simulink subsystem "Vehicle_Model"  (R2022b)
settings: Solver=VariableStepAuto  StartTime=0.0  StopTime=10.0  RelTol=1e-3
undefined symbols (not defined in the file): chassis, dZ, F0z, IMU_accel, IMU_gyro, IMU_mag, phi, powertrain, psi, sim, sus, suspension, theta, trn, veh, VEH, whl, X, Xdot, Y, Ydot, Z, Zdot
libraries: fl_lib x53, nesl_utility x15, vehdynlibtire x10, vehdynlibsuspension x8, EngineCoolingComponents_lib x5, autolibutils x5, sharedtransform x5, shared6dof x2, sensorgpslib x1, mspsensorlib x1, dspstat3 x1, SimscapeFluids_lib x1
(part 1 of 8)
settings Model: Creator=Inver  LastModifiedBy=Inver

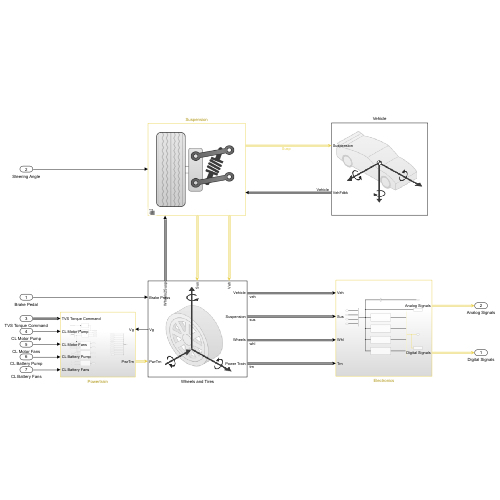
[thumbnail: Simulink's stored preview of the top-level diagram]
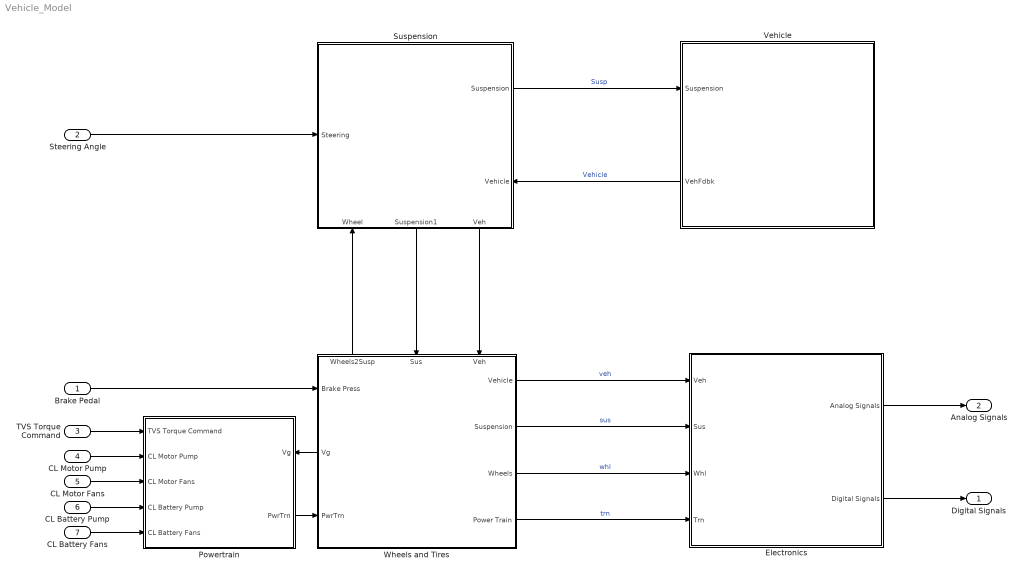
== system Vehicle_Model ==
  Brake Pedal : Inport
  Steering Angle : Inport  Port=2
  TVS Torque Command : Inport  Port=3
  CL Motor Pump : Inport  Port=4
  CL Motor Fans : Inport  Port=5
  CL Battery Pump : Inport  Port=6
  CL Battery Fans : Inport  Port=7
  Electronics : Subsystem
  Powertrain : Subsystem
      settings: PortSchema="{\"entries\":[{\"content\":{\"sides\":[{\"content\":{\"connectorIds\":[\"In1\",\"In2\",\"In3\",\"In4\",\"In5\"]},\"type\":\"ConnectorPlacement.EquallySpacedRectSide\",\"uuid\":\"895a90fc-946f-4344-af69-c005acf2f614\"},{\"content\":{\"connectorIds\":[\"In6\",\"Out1\"],\"side\":\"RIGHT\"},\"type\":\"ConnectorPlacement.EquallySpacedRectSide\",\"uuid\":\"931fcb49-b75e-480c-a4d6-2f82b080d057\"},{\"content\":{\"connectorIds\":[],\"side\":\"TOP\"},\"type\":\"ConnectorPlacement.EquallySpacedRectSide\",\"uuid\":\"d1b12b51-387e-4553-b5da-149d57232505\"}]},\"type\":\"ConnectorPlacement.EquallySpacedConnector\",\"uuid\":\"0cb2c3dd-4627-421c-9ed4-7e8c572a9937\"}],\"packageUris\":[\"http://schema.mathworks.com/mf0/Connector/R2020b\"],\"version\":\"1.0\"}"
  Suspension : Subsystem  Variant=on  VariantControlMode=label  LabelModeActiveChoice=1
      settings: PortSchema="{\"entries\":[{\"content\":{\"sides\":[{\"content\":{\"connectorIds\":[\"In1\"]},\"type\":\"ConnectorPlacement.EquallySpacedRectSide\",\"uuid\":\"d90bf910-501d-4dd1-a367-d76bd42ab174\"},{\"content\":{\"connectorIds\":[\"Out1\",\"In3\"],\"side\":\"RIGHT\"},\"type\":\"ConnectorPlacement.EquallySpacedRectSide\",\"uuid\":\"1fe7da07-1086-4d5e-8baf-d5d069455d6e\"},{\"content\":{\"connectorIds\":[],\"side\":\"TOP\"},\"type\":\"ConnectorPlacement.EquallySpacedRectSide\",\"uuid\":\"6ff63b9e-45bb-47e9-90cd-47f8e0815e57\"},{\"content\":{\"connectorIds\":[\"In2\",\"Out2\",\"Out3\"],\"side\":\"BOTTOM\"},\"type\":\"ConnectorPlacement.EquallySpacedRectSide\",\"uuid\":\"116c6de0-7bfa-4dc1-bfd0-57a2fffb3aa0\"}]},\"type\":\"ConnectorPlacement.EquallySpacedConnector\",\"uuid\":\"6475b998-12b0-4b0e-8a20-c379b8e08c7c\"}],\"packageUris\":[\"http://schema.mathworks.com/mf0/Connector/R2020b\"],\"version\":\"1.0\"}"
      mask Display:
      | switch str2num(get_param(gcb,'ActiveVariant'))
      |     case 1
      |         image('suspdw.png');
      |     case 2
      |         image([imread('suspindmap.png');imread('suspsamap.png')]);
      |     case 3
      |          image([imread('suspmacp.png');imread('suspsacoil.png')]);
      |     case 4
      |          image('suspmacp.png');
      |     case 5
      |          image('suspindmap.png');
      |     case 6
      |          image('suspkandc.png');
      | end
  Vehicle : Subsystem
      settings: PortSchema="{\"entries\":[{\"content\":{\"sides\":[{\"content\":{\"connectorIds\":[\"In1\",\"Out1\"]},\"type\":\"ConnectorPlacement.EquallySpacedRectSide\",\"uuid\":\"63fa377f-0583-4c60-bac7-9bd73dadd9a1\"},{\"content\":{\"connectorIds\":[],\"side\":\"RIGHT\"},\"type\":\"ConnectorPlacement.EquallySpacedRectSide\",\"uuid\":\"7f668e34-aa5e-4f2f-9be8-80fbb83ff2c8\"},{\"content\":{\"connectorIds\":[],\"side\":\"TOP\"},\"type\":\"ConnectorPlacement.EquallySpacedRectSide\",\"uuid\":\"511f439c-568f-45f1-9ff4-54e644eb8180\"}]},\"type\":\"ConnectorPlacement.EquallySpacedConnector\",\"uuid\":\"b54bf87e-fa06-468b-8fa9-38148d60ed3d\"}],\"packageUris\":[\"http://schema.mathworks.com/mf0/Connector/R2020b\"],\"version\":\"1.0\"}"
      mask Display: image('6dofcar.png');
  Wheels and Tires : Subsystem
      settings: PortSchema="{\"entries\":[{\"content\":{\"sides\":[{\"content\":{\"connectorIds\":[\"In1\",\"Out6\",\"In2\"]},\"type\":\"ConnectorPlacement.EquallySpacedRectSide\",\"uuid\":\"77263124-783e-4307-b979-a6212540af24\"},{\"content\":{\"connectorIds\":[\"Out1\",\"Out2\",\"Out3\",\"Out4\"],\"side\":\"RIGHT\"},\"type\":\"ConnectorPlacement.EquallySpacedRectSide\",\"uuid\":\"cb03b446-69c2-4dbf-929b-d33818acfe8b\"},{\"content\":{\"connectorIds\":[\"Out5\",\"In3\",\"In4\"],\"side\":\"TOP\"},\"type\":\"ConnectorPlacement.EquallySpacedRectSide\",\"uuid\":\"8e7e4023-62e5-48a8-8666-b4c8bb14cd01\"}]},\"type\":\"ConnectorPlacement.EquallySpacedConnector\",\"uuid\":\"1061f0db-ec8e-49bd-8d66-b4a53eaeacfa\"}],\"packageUris\":[\"http://schema.mathworks.com/mf0/Connector/R2020b\"],\"version\":\"1.0\"}"
      mask Display: image('wheel3dof.png')
  Digital Signals : Outport  PortDimensions={292}
  Analog Signals : Outport  Port=2  PortDimensions={292}
  wires:
  CL Motor Pump/1 -> Powertrain/2(CL Motor Pump)
  CL Motor Fans/1 -> Powertrain/3(CL Motor Fans)
  Wheels and Tires/1(Vehicle) -> Electronics/1(Veh)  "veh"
  Wheels and Tires/6(Vg) -> Powertrain/6(Vg)
  CL Battery Pump/1 -> Powertrain/4(CL Battery Pump)
  Electronics/2(Digital Signals) -> Digital Signals/1
  CL Battery Fans/1 -> Powertrain/5(CL Battery Fans)
  Vehicle/1(VehFdbk) -> Suspension/3(Vehicle)  "Vehicle"
  Suspension/2(Suspension1) -> Wheels and Tires/3(Sus)
  TVS Torque Command/1 -> Powertrain/1(TVS Torque Command)
  Steering Angle/1 -> Suspension/1(Steering)
  Electronics/1(Analog Signals) -> Analog Signals/1
  Wheels and Tires/5(Wheels2Susp) -> Suspension/2(Wheel)
  Brake Pedal/1 -> Wheels and Tires/1(Brake Press)
  Wheels and Tires/2(Suspension) -> Electronics/2(Sus)  "sus"
  Suspension/1(Suspension) -> Vehicle/1(Suspension)  "Susp"
  Suspension/3(Veh) -> Wheels and Tires/4(Veh)
  Powertrain/1(PwrTrn) -> Wheels and Tires/2(PwrTrn)
  Wheels and Tires/3(Wheels) -> Electronics/3(Whl)  "whl"
  Wheels and Tires/4(Power Train) -> Electronics/4(Trn)  "trn"

== system Vehicle_Model/Electronics ==
  Veh : Inport
  Sus : Inport  Port=2
  Whl : Inport  Port=3
  Trn : Inport  Port=4
  All Veh Info : BusCreator  Inputs=veh,sus,whl,trn
  Bus Selector2 : BusSelector  OutputSignals=veh.InertFrm.Cg.Disp,veh.InertFrm.Cg.Ang.psi,veh.BdyFrm.Cg.Vel,veh.BdyFrm.Cg.AngVel.r,sus.Sus.steering_angle,whl.TireFrame.Omega,whl.TireFrame.GndFz  OutputAsBus=on
  Cooling Sensors : Subsystem
  Corner Dynamics Sensors : Subsystem
  Digital SIgnals : BusCreator  Inputs=4
  Navigation Sensors : Subsystem
  Power Sensors : Subsystem
  To Workspace : ToWorkspace  VariableName=Digital_Signals  SaveFormat=Timeseries  SampleTime=-1
  To Workspace1 : ToWorkspace  VariableName=Vehicle_Signals  SaveFormat=Timeseries  SampleTime=-1
  Analog Signals : Outport
  Digital Signals : Outport  Port=2
  wires:
  Sus/1 -> All Veh Info/2
  Whl/1 -> All Veh Info/3
  Trn/1 -> All Veh Info/4
  Bus Selector2/1 -> Analog Signals/1
  Navigation Sensors/1(Navigation Sensors) -> Digital SIgnals/1  "Navigation Sensors"
  Power Sensors/1(Power Sensors) -> Digital SIgnals/2  "Power Sensors"
  Corner Dynamics Sensors/1(Corner Dynamics Sensors) -> Digital SIgnals/4  "Corner Dynamics Sensors"
  Digital SIgnals/1 -> Digital Signals/1, To Workspace/1  "Digital Signls"
  Cooling Sensors/1(Cooling Sensors) -> Digital SIgnals/3  "Cooling Sensors"
  All Veh Info/1 -> Bus Selector2/1, To Workspace1/1, Navigation Sensors/1(Analog Signals), Corner Dynamics Sensors/1(Analog Signals), Cooling Sensors/1(Analog Signals), Power Sensors/1(Analog Signals)
  Veh/1 -> All Veh Info/1  "veh"

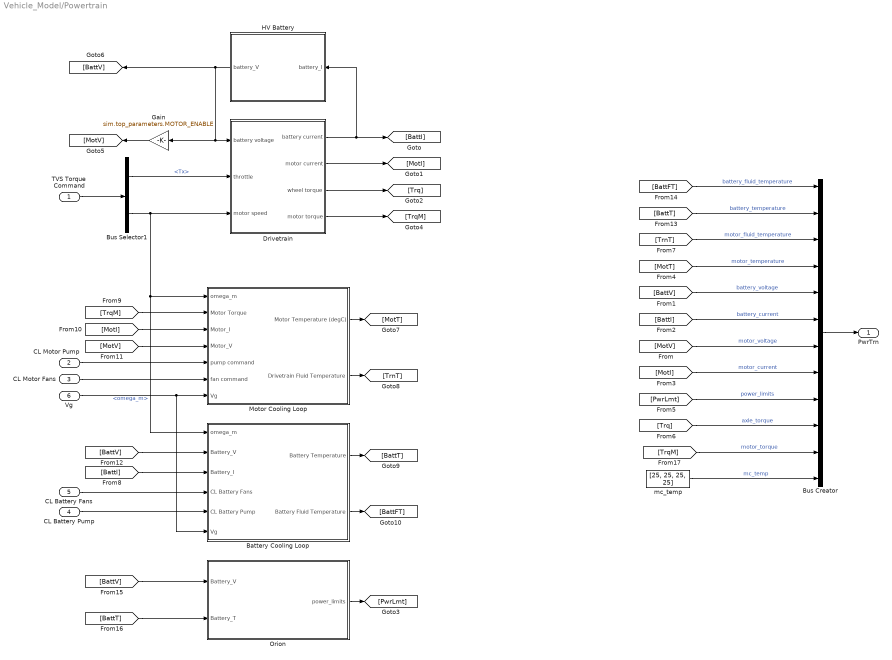
== system Vehicle_Model/Powertrain ==
  TVS Torque Command : Inport
  CL Motor Pump : Inport  Port=2
  CL Motor Fans : Inport  Port=3
  CL Battery Pump : Inport  Port=4
  CL Battery Fans : Inport  Port=5
  Vg : Inport  Port=6
  Battery Cooling Loop : Subsystem
  Bus Creator : BusCreator  Inputs=12
  Bus Selector1 : BusSelector  OutputSignals=Tx,omega_m
  Drivetrain : Subsystem
  Gain : Gain  Gain=sim.top_parameters.MOTOR_ENABLE
  HV Battery : Subsystem
  Motor Cooling Loop : Subsystem
  Orion : Subsystem
  mc_temp : Constant  Value=[25, 25, 25, 25]
  PwrTrn : Outport
  wires:
  Drivetrain/3(wheel torque) -> [Trq]
  [BattT] -> Orion/2(Battery_T)
  [Trq] -> Bus Creator/10  "axle_torque"
  [TrnT] -> Bus Creator/3  "motor_fluid_temperature"
  Vg/1 -> Motor Cooling Loop/7(Vg), Battery Cooling Loop/6(Vg)
  CL Battery Fans/1 -> Battery Cooling Loop/4(CL Battery Fans)
  [MotT] -> Bus Creator/4  "motor_temperature"
  Battery Cooling Loop/2(Battery Fluid Temperature) -> [BattFT]
  [BattI] -> Bus Creator/6  "battery_current"
  [MotI] -> Bus Creator/8  "motor_current"
  [MotV] -> Motor Cooling Loop/4(Motor_V)
  Motor Cooling Loop/2(Drivetrain Fluid Temperature) -> [TrnT]
  CL Battery Pump/1 -> Battery Cooling Loop/5(CL Battery Pump)
  Bus Selector1/2 -> Drivetrain/3(motor speed), Motor Cooling Loop/1(omega_m), Battery Cooling Loop/1(omega_m)  "<omega_m>"
  Bus Selector1/1 -> Drivetrain/2(throttle)  "<Tx>"
  CL Motor Pump/1 -> Motor Cooling Loop/5(pump command)
  Battery Cooling Loop/1(Battery Temperature) -> [BattT]
  [BattI] -> Battery Cooling Loop/3(Battery_I)
  [BattV] -> Orion/1(Battery_V)
  Motor Cooling Loop/1(Motor Temperature (degC)) -> [MotT]
  HV Battery/1(battery_V) -> [BattV], Gain/1, Drivetrain/1(battery voltage)
  [MotV] -> Bus Creator/7  "motor_voltage"
  [BattV] -> Bus Creator/5  "battery_voltage"
  [MotI] -> Motor Cooling Loop/3(Motor_I)
  [BattV] -> Battery Cooling Loop/2(Battery_V)
  [BattFT] -> Bus Creator/1  "battery_fluid_temperature"
  Drivetrain/1(battery current) -> HV Battery/1(battery_I), [BattI]
  Bus Creator/1 -> PwrTrn/1
  CL Motor Fans/1 -> Motor Cooling Loop/6(fan command)
  [PwrLmt] -> Bus Creator/9  "power_limits"
  [BattT] -> Bus Creator/2  "battery_temperature"
  Orion/1(power_limits) -> [PwrLmt]
  [TrqM] -> Motor Cooling Loop/2(Motor Torque)
  mc_temp/1 -> Bus Creator/12  "mc_temp"
  TVS Torque Command/1 -> Bus Selector1/1
  Drivetrain/4(motor torque) -> [TrqM]
  [TrqM] -> Bus Creator/11  "motor_torque"
  Drivetrain/2(motor current) -> [MotI]
  Gain/1 -> [MotV]

== system Vehicle_Model/Suspension ==
  Steering : Inport
  Wheel : Inport  Port=2
  Vehicle : Inport  Port=3
  Double Wishbone Suspension : Subsystem  VariantControl=1
      mask Display: image('suspdw.png');
  Independent Mapped Front Suspension Mapped Solid Axle Rear Suspension : Subsystem  VariantControl=2
      mask Display: image([imread('suspindmap.png');imread('suspsamap.png')]);
  Kinematics and Compliance Independent Suspension : Subsystem  VariantControl=6
      mask Display: image('suspkandc.png');
  MacPherson Front Suspension Solid Axle Rear Suspension : Subsystem  VariantControl=3
      mask Display: image([imread('suspmacp.png');imread('suspsacoil.png')]);
  MacPherson Suspension : Subsystem  VariantControl=4
      mask Display: image('suspmacp.png');
  Mapped Suspension : Subsystem  VariantControl=5
      mask Display: image('suspindmap.png');
  Suspension : Outport  VectorParamsAs1DForOutWhenUnconnected=off
  Suspension1 : Outport  Port=2  VectorParamsAs1DForOutWhenUnconnected=off
  Veh : Outport  Port=3  VectorParamsAs1DForOutWhenUnconnected=off

== system Vehicle_Model/Vehicle ==
  Suspension : Inport
  6DOF : Subsystem  VariantControl=1
  Constant : Constant  Value=[0 0 0]
  VehFdbk : Outport  VectorParamsAs1DForOutWhenUnconnected=off
  wires:
  6DOF/1(VehFdbk) -> VehFdbk/1  "VehFdbk"
  Constant/1 -> 6DOF/2(Wind)
  Suspension/1 -> 6DOF/1(Suspension)

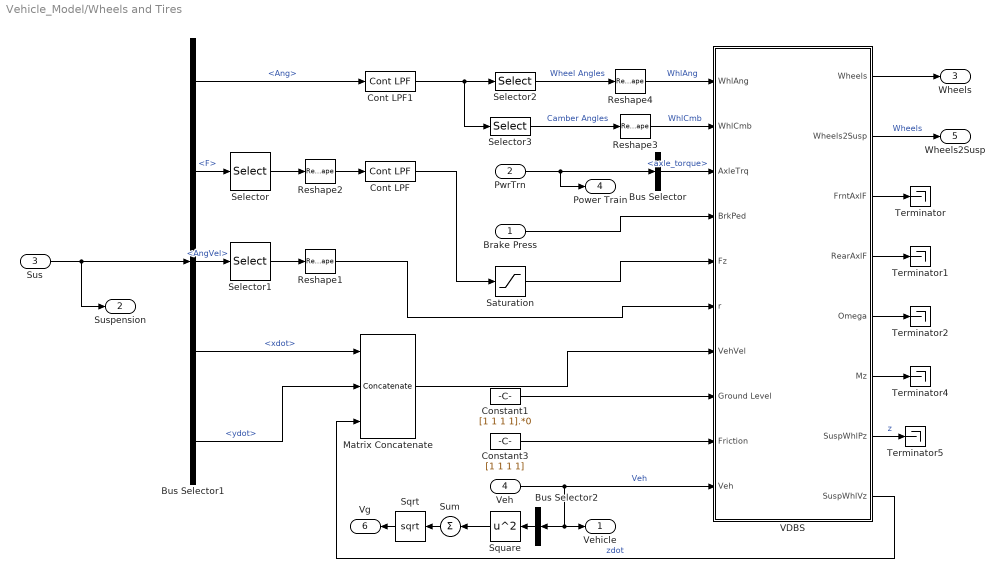
== system Vehicle_Model/Wheels and Tires ==
  Brake Press : Inport  Unit=Pa
  PwrTrn : Inport  Port=2
  Sus : Inport  Port=3
  Veh : Inport  Port=4
  Bus Selector : BusSelector  OutputSignals=axle_torque
  Bus Selector1 : BusSelector  OutputSignals=Whl.Ang,Whl.F,Whl.AngVel,Whl.xdot,Whl.ydot
  Bus Selector2 : BusSelector  OutputSignals=BdyFrm.Cg.Vel.xdot,BdyFrm.Cg.Vel.ydot  OutputAsBus=on
  Constant1 : Constant  Value=[1 1 1 1].*0
  Constant3 : Constant  Value=[1 1 1 1]
  Cont LPF : autolibutils/Cont LPF  wc=100*2*pi  AbsoluteTolerance=auto  aMode=2
  Cont LPF1 : autolibutils/Cont LPF  wc=100*2*pi  AbsoluteTolerance=auto  aMode=2
  Matrix Concatenate : Concatenate  NumInputs=3  Mode=Multidimensional array
  Reshape{1..4} (4 alike) : Reshape
  Saturation : Saturate  UpperLimit=inf  LowerLimit=-10*9.81*2000  ZeroCross=off
  Selector : Selector  NumberOfDimensions=2  InputPortWidth=3  IndexOptions=Index vector (dialog),Select all  Indices=[3],1  OutputSizes=1,1
  Selector1 : Selector  NumberOfDimensions=2  InputPortWidth=1  IndexOptions=Index vector (dialog),Select all  Indices=[3],1  OutputSizes=1,1
  Selector2 : Selector  NumberOfDimensions=2  InputPortWidth=3  IndexOptions=Index vector (dialog),Select all  Indices=3,1  OutputSizes=1,1
  Selector3 : Selector  NumberOfDimensions=2  InputPortWidth=3  IndexOptions=Index vector (dialog),Select all  Indices=1,1  OutputSizes=1,1
  Sqrt : Sqrt
  Square : Math  Operator=square
  Sum : Sum  Inputs=+
  Terminator{,1..2,4..5} (5 alike) : Terminator
  VDBS : Subsystem  VariantControl=0
  Vehicle : Outport  VectorParamsAs1DForOutWhenUnconnected=off
  Suspension : Outport  Port=2  VectorParamsAs1DForOutWhenUnconnected=off
  Wheels : Outport  Port=3  VectorParamsAs1DForOutWhenUnconnected=off
  Power Train : Outport  Port=4  VectorParamsAs1DForOutWhenUnconnected=off
  Wheels2Susp : Outport  Port=5  VectorParamsAs1DForOutWhenUnconnected=off
  Vg : Outport  Port=6  VectorParamsAs1DForOutWhenUnconnected=off
  wires:
  Bus Selector1/2 -> Selector/1  "<F>"
  VDBS/3(FrntAxlF) -> Terminator/1
  VDBS/4(RearAxlF) -> Terminator1/1
  VDBS/6(Mz) -> Terminator4/1
  Selector1/1 -> Reshape1/1
  Matrix Concatenate/1 -> VDBS/7(VehVel)
  PwrTrn/1 -> Power Train/1, Bus Selector/1
  Reshape4/1 -> VDBS/1(WhlAng)  "WhlAng"
  Reshape3/1 -> VDBS/2(WhlCmb)  "WhlCmb"
  Selector/1 -> Reshape2/1
  Saturation/1 -> VDBS/5(Fz)
  Constant1/1 -> VDBS/8(Ground Level)
  VDBS/8(SuspWhlVz) -> Matrix Concatenate/3  "zdot"
  Bus Selector1/1 -> Cont LPF1/1  "<Ang>"
  Selector3/1 -> Reshape3/1  "Camber Angles"
  Sus/1 -> Suspension/1, Bus Selector1/1
  Bus Selector1/4 -> Matrix Concatenate/1  "<xdot>"
  Bus Selector1/5 -> Matrix Concatenate/2  "<ydot>"
  VDBS/7(SuspWhlPz) -> Terminator5/1  "z"
  Reshape2/1 -> Cont LPF/1
  Bus Selector1/3 -> Selector1/1  "<AngVel>"
  Reshape1/1 -> VDBS/6(r)
  Brake Press/1 -> VDBS/4(BrkPed)
  Constant3/1 -> VDBS/9(Friction)
  Cont LPF/1 -> Saturation/1
  Cont LPF1/1 -> Selector3/1, Selector2/1
  Selector2/1 -> Reshape4/1  "Wheel Angles"
  Veh/1 -> Vehicle/1, Bus Selector2/1, VDBS/10(Veh)  "Veh"
  VDBS/2(Wheels2Susp) -> Wheels2Susp/1  "Wheels"
  VDBS/1(Wheels) -> Wheels/1
  Bus Selector/1 -> VDBS/3(AxleTrq)  "<axle_torque>"
  VDBS/5(Omega) -> Terminator2/1
  Bus Selector2/1 -> Square/1
  Square/1 -> Sum/1
  Sum/1 -> Sqrt/1
  Sqrt/1 -> Vg/1

== system Vehicle_Model/Electronics/Cooling Sensors ==
  Analog Signals : Inport
  Bus Creator9 : BusCreator  Inputs=5
  Bus Selector : BusSelector  OutputSignals=trn.motor_temperature,trn.mc_temp,trn.motor_fluid_temperature,trn.battery_temperature,trn.battery_fluid_temperature
  Delay1 : Delay  InitialCondition=[1 1; 1 1; 1 1; 1 1].*sim.IC.motor_T_IC
  Delay11 : Delay  InitialCondition=[1 1; 1 1; 1 1; 1 1].*sim.IC.motor_T_IC
  Delay12 : Delay  InitialCondition=[1 1; 1 1].*sim.IC.motor_FT_IC
  Delay13 : Delay  InitialCondition=[1 1].*sim.IC.battery_T_IC
  Delay14 : Delay  InitialCondition=[1 1].*sim.IC.battery_FT_IC
  Rate Transition1 : RateTransition  InitialCondition=[1 1].*sim.IC.motor_FT_IC  OutPortSampleTime=0
  Rate Transition2 : RateTransition  InitialCondition=sim.IC.battery_T_IC  OutPortSampleTime=0
  Rate Transition3 : RateTransition  InitialCondition=sim.IC.battery_FT_IC  OutPortSampleTime=0
  Saturation10 : Saturate  UpperLimit=sim.range.MOTOR_TEMPERATURE_MAX  LowerLimit=sim.range.MOTOR_TEMPERATURE_MIN
  Saturation11 : Saturate  UpperLimit=sim.range.BATTERY_TEMPERATURE_MAX  LowerLimit=sim.range.BATTERY_TEMPERATURE_MIN
  Saturation12 : Saturate  UpperLimit=sim.range.BATTERY_TEMPERATURE_MAX  LowerLimit=sim.range.BATTERY_TEMPERATURE_MIN
  Saturation18 : Saturate  UpperLimit=sim.range.MOTOR_TEMPERATURE_MAX  LowerLimit=sim.range.MOTOR_TEMPERATURE_MIN
  Saturation21 : Saturate  UpperLimit=sim.range.MOTOR_TEMPERATURE_MAX  LowerLimit=sim.range.MOTOR_TEMPERATURE_MIN
  Zero-Order Hold{1,11..14} (5 alike) : ZeroOrderHold  SampleTime=sim.timing.duplicate
  Cooling Sensors : Outport
  wires:
  Delay1/1 -> Saturation21/1
  Saturation21/1 -> Bus Creator9/2  "mc_T"
  Bus Selector/2 -> Zero-Order Hold1/1  "<mc_temp>"
  Zero-Order Hold1/1 -> Delay1/1
  Delay14/1 -> Saturation12/1
  Delay11/1 -> Saturation18/1
  Delay12/1 -> Saturation10/1
  Saturation12/1 -> Bus Creator9/5  "batt_FT"
  Zero-Order Hold12/1 -> Delay12/1
  Zero-Order Hold14/1 -> Delay14/1
  Bus Selector/4 -> Rate Transition2/1  "<battery_temperature>"
  Zero-Order Hold11/1 -> Delay11/1
  Saturation18/1 -> Bus Creator9/1  "motor_T"
  Zero-Order Hold13/1 -> Delay13/1
  Bus Selector/3 -> Rate Transition1/1  "<motor_fluid_temperature>"
  Saturation11/1 -> Bus Creator9/4  "batt_T"
  Saturation10/1 -> Bus Creator9/3  "motor_FT"
  Delay13/1 -> Saturation11/1
  Bus Selector/1 -> Zero-Order Hold11/1  "<motor_temperature>"
  Bus Selector/5 -> Rate Transition3/1  "<battery_fluid_temperature>"
  Bus Creator9/1 -> Cooling Sensors/1
  Rate Transition1/1 -> Zero-Order Hold12/1  "motor_fluid_temperature"
  Rate Transition2/1 -> Zero-Order Hold13/1  "battery_temperature"
  Rate Transition3/1 -> Zero-Order Hold14/1  "battery_fluid_temperature"
  Analog Signals/1 -> Bus Selector/1

== system Vehicle_Model/Electronics/Corner Dynamics Sensors ==
  Analog Signals : Inport
  Bus Creator10 : BusCreator  Inputs=4
  Bus Selector : BusSelector  OutputSignals=whl.TireFrame.Omega,sus.Sus.steering_angle,sus.Sus.shock_length,whl.TireFrame.GndFz
  Delay15 : Delay  InitialCondition=ones(1, 4, 2).*sim.IC.omega_IC
  Delay16 : Delay  InitialCondition=[1 1].*sim.IC.theta_IC
  Delay17 : Delay  InitialCondition=[1 1; 1 1; 1 1; 1 1].*sim.IC.shock_length_IC
  Delay18 : Delay  InitialCondition=[1 1; 1 1; 1 1; 1 1].*sim.IC.Fz_IC
  Saturation15 : Saturate  UpperLimit=sim.range.SHOCK_LENGTH_MAX  LowerLimit=sim.range.SHOCK_LENGTH_MIN
  Saturation16 : Saturate  UpperLimit=sim.range.OMEGA_MAX  LowerLimit=sim.range.OMEGA_MIN
  Saturation17 : Saturate  UpperLimit=sim.range.FZ_MAX  LowerLimit=sim.range.FZ_MIN
  Saturation3 : Saturate  UpperLimit=sim.range.CENTER_STEER_ANGLE_MAX  LowerLimit=-sim.range.CENTER_STEER_ANGLE_MAX
  Transpose : Math  Operator=transpose
  Zero-Order Hold{15..18} (4 alike) : ZeroOrderHold  SampleTime=sim.timing.duplicate
  Corner Dynamics Sensors : Outport
  wires:
  Transpose/1 -> Zero-Order Hold15/1  "omega"
  Bus Selector/1 -> Transpose/1  "<Omega>"
  Zero-Order Hold18/1 -> Delay18/1
  Delay18/1 -> Saturation17/1
  Zero-Order Hold15/1 -> Delay15/1
  Zero-Order Hold16/1 -> Delay16/1
  Saturation17/1 -> Bus Creator10/4  "FZ"
  Saturation3/1 -> Bus Creator10/2  "theta"
  Bus Selector/3 -> Zero-Order Hold17/1  "<shock_length>"
  Saturation15/1 -> Bus Creator10/3  "shock_L"
  Saturation16/1 -> Bus Creator10/1  "omega"
  Bus Selector/4 -> Zero-Order Hold18/1  "<GndFz>"
  Delay16/1 -> Saturation3/1
  Bus Selector/2 -> Zero-Order Hold16/1  "<steering_angle>"
  Delay17/1 -> Saturation15/1
  Delay15/1 -> Saturation16/1
  Zero-Order Hold17/1 -> Delay17/1
  Bus Creator10/1 -> Corner Dynamics Sensors/1
  Analog Signals/1 -> Bus Selector/1

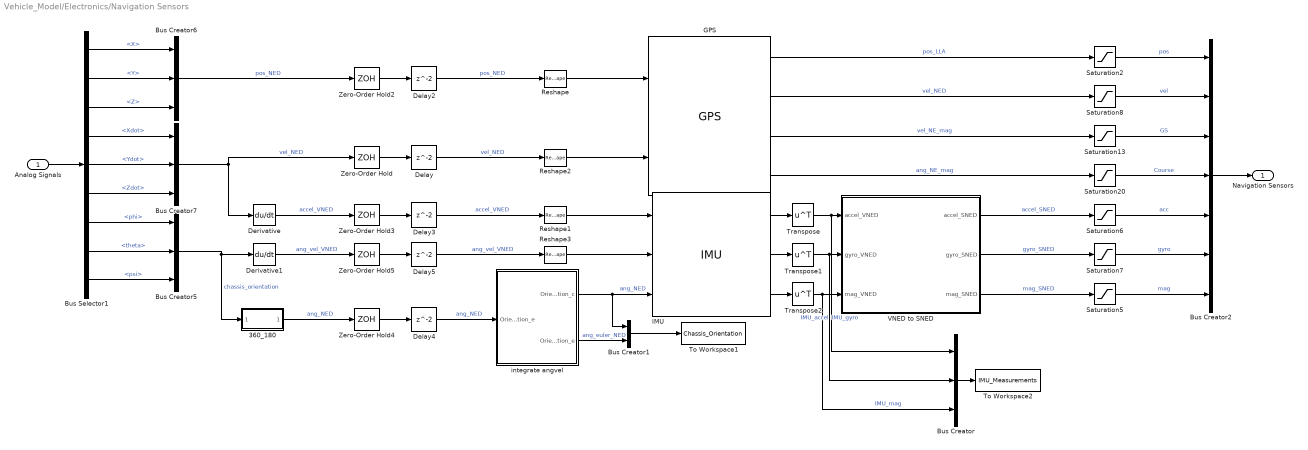
== system Vehicle_Model/Electronics/Navigation Sensors ==
  Analog Signals : Inport
  360_180 : Subsystem
  Bus Creator : BusCreator  Inputs=IMU_accel,IMU_gyro,IMU_mag
  Bus Creator1 : BusCreator  Inputs=2
  Bus Creator2 : BusCreator  Inputs=7
  Bus Creator5 : BusCreator  Inputs=phi,theta,psi
  Bus Creator6 : BusCreator  Inputs=X,Y,Z
  Bus Creator7 : BusCreator  Inputs=Xdot,Ydot,Zdot
  Bus Selector1 : BusSelector  OutputSignals=veh.InertFrm.Cg.Disp.X,veh.InertFrm.Cg.Disp.Y,veh.InertFrm.Cg.Disp.Z,veh.InertFrm.Cg.Vel.Xdot,veh.InertFrm.Cg.Vel.Ydot,veh.InertFrm.Cg.Vel.Zdot,veh.InertFrm.Cg.Ang.phi,veh.InertFrm.Cg.Ang.theta,veh.InertFrm.Cg.Ang.psi
  Delay : Delay  InitialCondition=([1;1]*sim.IC.vel_IC)'
  Delay2 : Delay  InitialCondition=[1 1; 1 1; 1 1].*sim.IC.pos_IC
  Delay3 : Delay  InitialCondition=[1 1; 1 1; 1 1].*sim.IC.acc_IC
  Delay4 : Delay  InitialCondition=[1 1; 1 1; 1 1].*sim.IC.ang_IC
  Delay5 : Delay  InitialCondition=[1 1; 1 1; 1 1].*sim.IC.ang_vel_IC
  Derivative : Derivative
  Derivative1 : Derivative
  GPS : sensorgpslib/GPS  DispRefFrame=NED  PositionInputFormat=Local  ReferenceLocation=sim.IC.location_lla_IC  HorizontalPositionAccuracy=sensor.gps.GPS_Z_ACCURACY  VerticalPositionAccuracy=sensor.gps.GPS_XY_ACCURACY  VelocityAccuracy=sensor.gps.GPS_V_ACCURACY  DecayFactor=sensor.gps.GPS_NOISE_FACTOR  SeedDouble=sensor.gps.r_GPS  SimulateUsing=Interpreted execution
      settings: LibrarySourceBlock=mspsensorlib/GPS
  IMU : mspsensorlib/IMU  DispRefFrame=NED  Temperature=25  MagneticFieldNED=sim.IC.mag_field_IC  MagneticFieldENU=[ -2.4169, 27.5550, 16.0849 ]  SeedDouble=sensor.imu.r_IMU  SimulateUsing=Interpreted execution  AccelParamsMeasurementRange=sensor.imu.ACC_MAX  AccelParamsResolution=sensor.imu.ACC_RES  AccelParamsConstantBias=sensor.imu.ACC_BIAS  AccelParamsAxesMisalignment=sensor.imu.ACC_SKEW  AccelParamsNoiseDensity=sensor.imu.ACC_VEL_WALK  AccelParamsBiasInstability=sensor.imu.ACC_BIAS_INSTABILITY  AccelParamsRandomWalk=sensor.imu.ACC_WALK  AccelParamsTemperatureBias=sensor.imu.ACC_T_BIAS  AccelParamsTemperatureScaleFactor=sensor.imu.ACC_T_SCALE  GyroParamsMeasurementRange=sensor.imu.GYR_MAX  GyroParamsResolution=sensor.imu.GYR_RES  GyroParamsConstantBias=sensor.imu.GYR_BIAS  GyroParamsAxesMisalignment=sensor.imu.GYR_SKEW  GyroParamsAccelerationBias=sensor.imu.GYR_ACC_BIAS  GyroParamsNoiseDensity=sensor.imu.GYR_ANG_WALK  GyroParamsBiasInstability=sensor.imu.GYR_BIAS_INSTABILITY  GyroParamsRandomWalk=sensor.imu.GYR_WALK  GyroParamsTemperatureBias=sensor.imu.GYR_T_BIAS  GyroParamsTemperatureScaleFactor=sensor.imu.GYR_T_SCALE  MagParamsMeasurementRange=sensor.imu.MAG_MAX  MagParamsResolution=sensor.imu.MAG_RES  MagParamsConstantBias=sensor.imu.MAG_BIAS  MagParamsAxesMisalignment=sensor.imu.MAG_SKEW  MagParamsNoiseDensity=sensor.imu.MAG_WHITE  MagParamsBiasInstability=sensor.imu.MAG_BIAS_INSTABILITY  MagParamsRandomWalk=sensor.imu.MAG_WALK  MagParamsTemperatureBias=sensor.imu.MAG_T_BIAS  MagParamsTemperatureScaleFactor=sensor.imu.MAG_T_SCALE
  Reshape{,1..3} (4 alike) : Reshape  OutputDimensionality=Row vector (2-D)
  Saturation13 : Saturate  UpperLimit=sim.range.VELOCITY_MAX  LowerLimit=-sim.range.VELOCITY_MAX
  Saturation2 : Saturate  UpperLimit=inf  LowerLimit=-inf
  Saturation20 : Saturate  UpperLimit=sim.range.ORIENTATION_MAX  LowerLimit=-sim.range.ORIENTATION_MAX
  Saturation5 : Saturate  UpperLimit=sim.range.MAG_MAX  LowerLimit=-sim.range.MAG_MAX
  Saturation6 : Saturate  UpperLimit=sim.range.ACCELERATION_MAX  LowerLimit=-sim.range.ACCELERATION_MAX
  Saturation7 : Saturate  UpperLimit=sim.range.YAW_MAX  LowerLimit=-sim.range.YAW_MAX
  Saturation8 : Saturate  UpperLimit=sim.range.VELOCITY_MAX  LowerLimit=-sim.range.VELOCITY_MAX
  To Workspace1 : ToWorkspace  VariableName=Chassis_Orientation  SaveFormat=Timeseries  SampleTime=-1
  To Workspace2 : ToWorkspace  VariableName=IMU_Measurements  SaveFormat=Timeseries  SampleTime=-1
  Transpose : Math  Operator=transpose
  Transpose1 : Math  Operator=transpose
  Transpose2 : Math  Operator=transpose
  VNED to SNED : MATLAB Function  TreatAsAtomicUnit=on
  Zero-Order Hold{,2..5} (5 alike) : ZeroOrderHold  SampleTime=sim.timing.duplicate
  integrate angvel : MATLAB Function  TreatAsAtomicUnit=on
  Navigation Sensors : Outport
  wires:
  Delay5/1 -> Reshape3/1  "ang_vel_VNED"
  Delay/1 -> Reshape2/1  "vel_NED"
  Delay3/1 -> Reshape1/1  "accel_VNED"
  Delay2/1 -> Reshape/1  "pos_NED"
  integrate angvel/1(Orientation_c) -> Bus Creator1/1, IMU/3  "ang_NED"
  GPS/4 -> Saturation20/1  "ang_NE_mag"
  GPS/3 -> Saturation13/1  "vel_NE_mag"
  GPS/2 -> Saturation8/1  "vel_NED"
  GPS/1 -> Saturation2/1  "pos_LLA"
  VNED to SNED/2(gyro_SNED) -> Saturation7/1  "gyro_SNED"
  VNED to SNED/1(accel_SNED) -> Saturation6/1  "accel_SNED"
  VNED to SNED/3(mag_SNED) -> Saturation5/1  "mag_SNED"
  Delay4/1 -> integrate angvel/1("Orientation_e ")  "ang_NED"
  Transpose2/1 -> Bus Creator/3, VNED to SNED/3(mag_VNED)  "IMU_mag"
  Transpose1/1 -> Bus Creator/2, VNED to SNED/2(gyro_VNED)  "IMU_gyro"
  Transpose/1 -> Bus Creator/1, VNED to SNED/1(accel_VNED)  "IMU_accel"
  IMU/3 -> Transpose2/1
  IMU/1 -> Transpose/1
  IMU/2 -> Transpose1/1
  Bus Creator/1 -> To Workspace2/1
  Bus Creator1/1 -> To Workspace1/1
  integrate angvel/2(Orientation_e) -> Bus Creator1/2  "ang_euler_NED"
  Zero-Order Hold/1 -> Delay/1
  Bus Creator7/1 -> Zero-Order Hold/1, Derivative/1  "vel_NED"
  Zero-Order Hold2/1 -> Delay2/1
  Bus Creator6/1 -> Zero-Order Hold2/1  "pos_NED"
  Zero-Order Hold3/1 -> Delay3/1
  Derivative/1 -> Zero-Order Hold3/1  "accel_VNED"
  Zero-Order Hold5/1 -> Delay5/1
  Derivative1/1 -> Zero-Order Hold5/1  "ang_vel_VNED"
  Zero-Order Hold4/1 -> Delay4/1
  360_180/1(psi_rev) -> Zero-Order Hold4/1  "ang_NED"
  Saturation2/1 -> Bus Creator2/1  "pos"
  Saturation13/1 -> Bus Creator2/3  "GS"
  Saturation6/1 -> Bus Creator2/5  "acc"
  Saturation20/1 -> Bus Creator2/4  "Course"
  Saturation5/1 -> Bus Creator2/7  "mag"
  Saturation8/1 -> Bus Creator2/2  "vel"
  Saturation7/1 -> Bus Creator2/6  "gyro"
  Bus Creator2/1 -> Navigation Sensors/1
  Bus Selector1/1 -> Bus Creator6/1  "<X>"
  Bus Selector1/8 -> Bus Creator5/2  "<theta>"
  Bus Selector1/2 -> Bus Creator6/2  "<Y>"
  Bus Selector1/6 -> Bus Creator7/3  "<Zdot>"
  Bus Selector1/5 -> Bus Creator7/2  "<Ydot>"
  Bus Selector1/4 -> Bus Creator7/1  "<Xdot>"
  Bus Selector1/7 -> Bus Creator5/1  "<phi>"
  Bus Creator5/1 -> 360_180/1(<psi>), Derivative1/1  "chassis_orientation"
  Bus Selector1/3 -> Bus Creator6/3  "<Z>"
  Bus Selector1/9 -> Bus Creator5/3  "<psi>"
  Analog Signals/1 -> Bus Selector1/1
  Reshape/1 -> GPS/1
  Reshape1/1 -> IMU/1
  Reshape2/1 -> GPS/2
  Reshape3/1 -> IMU/2

== system Vehicle_Model/Electronics/Power Sensors ==
  Analog Signals : Inport
  Bus Creator8 : BusCreator  Inputs=5
  Bus Selector : BusSelector  OutputSignals=trn.battery_voltage,trn.battery_current,trn.motor_voltage,trn.motor_current,trn.power_limits
  Delay10 : Delay  InitialCondition=[sim.IC.dcl_IC; sim.IC.ccl_IC]*[1 1]
  Delay6 : Delay  InitialCondition=[1 1].*sim.IC.battery_voltage_IC
  Delay7 : Delay  InitialCondition=[1 1].*sim.IC.battery_current_IC
  Delay8 : Delay  InitialCondition=ones(1, 4, 2).*sim.IC.motor_voltage_IC
  Delay9 : Delay  InitialCondition=ones(1, 4, 2).*sim.IC.motor_current_IC
  Saturation1 : Saturate  UpperLimit=sim.range.BATTERY_CURRENT_MAX  LowerLimit=sim.range.BATTERY_CURRENT_MIN
  Saturation14 : Saturate  UpperLimit=sim.range.DCL_MAX  LowerLimit=sim.range.DCL_MIN
  Saturation19 : Saturate  UpperLimit=sim.range.BATTERY_VOLTAGE_MAX  LowerLimit=sim.range.BATTERY_VOLTAGE_MIN
  Saturation4 : Saturate  UpperLimit=sim.range.MOTOR_VOLTAGE_MAX  LowerLimit=sim.range.MOTOR_VOLTAGE_MIN
  Saturation9 : Saturate  UpperLimit=sim.range.MOTOR_CURRENT_MAX  LowerLimit=sim.range.MOTOR_CURRENT_MIN
  Zero-Order Hold{6..10} (5 alike) : ZeroOrderHold  SampleTime=sim.timing.duplicate
  Power Sensors : Outport
  wires:
  Zero-Order Hold6/1 -> Delay6/1
  Delay6/1 -> Saturation19/1
  Bus Selector/1 -> Zero-Order Hold6/1  "<battery_voltage>"
  Delay7/1 -> Saturation1/1
  Zero-Order Hold7/1 -> Delay7/1
  Bus Selector/2 -> Zero-Order Hold7/1  "<battery_current>"
  Delay8/1 -> Saturation4/1
  Zero-Order Hold8/1 -> Delay8/1
  Bus Selector/3 -> Zero-Order Hold8/1  "<motor_voltage>"
  Delay9/1 -> Saturation9/1
  Zero-Order Hold9/1 -> Delay9/1
  Bus Selector/4 -> Zero-Order Hold9/1  "<motor_current>"
  Zero-Order Hold10/1 -> Delay10/1
  Delay10/1 -> Saturation14/1
  Bus Selector/5 -> Zero-Order Hold10/1  "<power_limits>"
  Saturation19/1 -> Bus Creator8/1  "batt_V"
  Saturation1/1 -> Bus Creator8/2  "batt_I"
  Saturation9/1 -> Bus Creator8/4  "motor_I"
  Saturation4/1 -> Bus Creator8/3  "motor_V"
  Saturation14/1 -> Bus Creator8/5  "pwr_lmt"
  Bus Creator8/1 -> Power Sensors/1
  Analog Signals/1 -> Bus Selector/1

== system Vehicle_Model/Powertrain/Battery Cooling Loop ==
  omega_m : Inport
  Battery_V : Inport  Port=2
  Battery_I : Inport  Port=3
  CL Battery Fans : Inport  Port=4
  CL Battery Pump : Inport  Port=5
  Vg : Inport  Port=6
  Battery Temperature : Outport
  Battery Fluid Temperature : Outport  Port=2

== system Vehicle_Model/Powertrain/Drivetrain ==
  battery voltage : Inport
  throttle : Inport  Port=2
  motor speed : Inport  Port=3
  1-D Lookup Table : Lookup_n-D  NumberOfTableDimensions=1  LookupTableObject=''  BreakpointsForDimension1=powertrain.motor.speed_bp  BreakpointsForDimension1FirstPoint=10  BreakpointsForDimension2FirstPoint=10  BreakpointsForDimension1Spacing=12  BreakpointsForDimension2Spacing=12  BeginIndexSearchUsingPreviousIndexResult=on  Table=powertrain.motor.max_torque_table  ExtrapMethod=Clip  DiagnosticForOutOfRangeInput=Error  InternalRulePriority=Speed  RndMeth=Simplest
  1-D Lookup Table1 : Lookup_n-D  NumberOfTableDimensions=1  LookupTableObject=''  BreakpointsForDimension1=powertrain.motor.speed_bp  BreakpointsForDimension1FirstPoint=10  BreakpointsForDimension2FirstPoint=10  BreakpointsForDimension1Spacing=12  BreakpointsForDimension2Spacing=12  BeginIndexSearchUsingPreviousIndexResult=on  Table=powertrain.motor.max_current_table  ExtrapMethod=Clip  DiagnosticForOutOfRangeInput=Error  InternalRulePriority=Speed  RndMeth=Simplest
  Gain : Gain  Gain=sim.top_parameters.MOTOR_ENABLE
  Gain1 : Gain  Gain=powertrain.gearbox.gr.*powertrain.gearbox.ge
  Gain2 : Gain  Gain=sim.top_parameters.MOTOR_ENABLE
  Mean : dspstat3/Mean  run=off  InputProcessing=Columns as channels (frame based)  reset_popup=None  directionMode=Entire input  dimension=1  roiEnable=off  roiType=Rectangles  roiPortion=Entire ROI  roiOutput=Individual statistics for each ROI  roiFlag=off  roundingMode=Floor  overflowMode=off  outputDataTypeStr=Inherit: Same as accumulator  outputMin=[]  outputMax=[]  outputLastDataTypeStr=Inherit: Same as accumulator
  Product : Product
  Product1 : Product
  Sum : Sum  Inputs=+
  Terminator : Terminator
  battery current : Outport
  motor current : Outport  Port=2
  wheel torque : Outport  Port=3
  motor torque : Outport  Port=4
  wires:
  1-D Lookup Table/1 -> Gain/1
  motor speed/1 -> 1-D Lookup Table1/1, Mean/1
  Product/1 -> motor torque/1, Gain1/1
  throttle/1 -> Product/1, Product1/1
  Gain/1 -> Product/2
  Gain1/1 -> wheel torque/1
  Sum/1 -> battery current/1
  battery voltage/1 -> Terminator/1
  Mean/1 -> 1-D Lookup Table/1
  1-D Lookup Table1/1 -> Gain2/1
  Gain2/1 -> Product1/2
  Product1/1 -> motor current/1, Sum/1

== system Vehicle_Model/Powertrain/HV Battery ==
  battery_I : Inport
  1-D Lookup Table : Lookup_n-D  NumberOfTableDimensions=1  BreakpointsForDimension1=powertrain.battery.SOC  Table=powertrain.battery.Em  InternalRulePriority=Speed  RndMeth=Simplest
  Constant1 : Constant  Value=sim.IC.SOC_IC
  Gain : Gain  Gain=1/(3600*powertrain.battery.Np*powertrain.battery.Ah)
  Gain1 : Gain  Gain=powertrain.battery.Ns
  Gain2 : Gain  Gain=powertrain.battery.R
  Integrator : Integrator
  Sum1 : Sum  Inputs=|+-
  Sum2 : Sum  Inputs=|+-
  battery_V : Outport
  wires:
  Gain/1 -> Sum1/2
  Constant1/1 -> Sum1/1
  Gain2/1 -> Sum2/2
  Integrator/1 -> Gain/1
  Sum2/1 -> battery_V/1
  battery_I/1 -> Gain2/1, Integrator/1
  Sum1/1 -> 1-D Lookup Table/1  "SOC"
  1-D Lookup Table/1 -> Gain1/1
  Gain1/1 -> Sum2/1
